simulink model "clustercar8"  (R2016a)
settings: Solver=ode45  StartTime=0.0  StopTime=10.0  MaxStep=0.001  RelTol=1e-3
InitFcn:
  | clc;
  | clear;
  | R = 1/2;
  | L = 1;
  | L1 = [-1 0 1;1 -1 0;0 1 -1];
  | 
  | gammar = 0.75;
  | L1 = [L1,gammar*L1];
  | Vx = [0 0 0]';
  | Vy = [0 0 0];
  | Xend = [3 4 5]';
  | Yend = [3 4 5]';
StopFcn:
  | hold off
  | plot(xx(:,1),xx(:,2),'r',xx(:,3),xx(:,4),'b',xx(:,5),xx(:,6),'g');
  | hold on
  | grid on
  | plot(ss(:,1),ss(:,4),'k--',ss(:,2),ss(:,5),'c--',ss(:,3),ss(:,6),'m--');
libraries: simulink x3
settings Model: Creator=Administrator  LastModifiedBy=Administrator

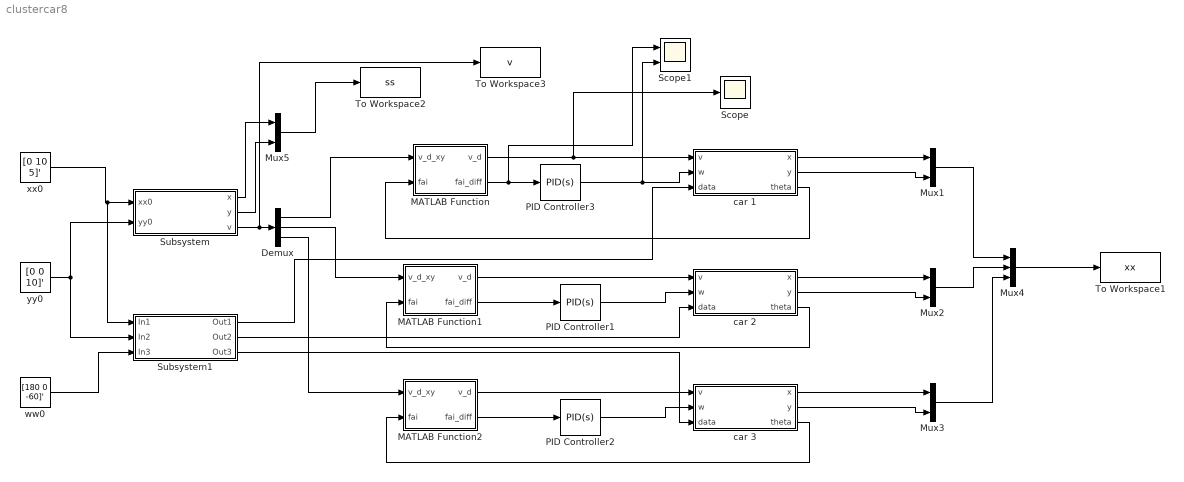
== system clustercar8 ==
  Demux : Demux  Outputs=3
  MATLAB Function : MATLAB Function  TreatAsAtomicUnit=on
  MATLAB Function1 : MATLAB Function  TreatAsAtomicUnit=on
  MATLAB Function2 : MATLAB Function  TreatAsAtomicUnit=on
  Mux{1..3,5} (4 alike) : Mux  Inputs=2
  Mux4 : Mux  Inputs=3
  PID Controller1 : simulink/Continuous/PID Controller  Controller=PID  TimeDomain=Continuous-time  SampleTime=-1  IntegratorMethod=Forward Euler  FilterMethod=Forward Euler  Form=Parallel  UseFilter=on  ControllerParametersSource=internal  P=100  I=10  D=0.01  N=100  InitialConditionSource=internal  InitialConditionForIntegrator=0  InitialConditionForFilter=0  ExternalReset=none  LimitOutput=off  UpperSaturationLimit=inf  LowerSaturationLimit=-inf  LinearizeAsGain=on  AntiWindupMode=none  Kb=1  TrackingMode=off  Kt=1  PParamMin=[]  PParamMax=[]  IParamMin=[]  IParamMax=[]  DParamMin=[]  DParamMax=[]  NParamMin=[]  NParamMax=[]  KbParamMin=[]  KbParamMax=[]  KtParamMin=[]  KtParamMax=[]  POutMin=[]  POutMax=[]  IOutMin=[]  IOutMax=[]  DOutMin=[]  DOutMax=[]  NOutMin=[]  NOutMax=[]  KbOutMin=[]  KbOutMax=[]  KtOutMin=[]  KtOutMax=[]  IntegratorOutMin=[]  IntegratorOutMax=[]  FilterOutMin=[]  FilterOutMax=[]  SumOutMin=[]  SumOutMax=[]  SumI1OutMin=[]  SumI1OutMax=[]  SumI2OutMin=[]  SumI2OutMax=[]  SumI3OutMin=[]  SumI3OutMax=[]  SumDOutMin=[]  SumDOutMax=[]  SaturationOutMin=[]  SaturationOutMax=[]  IntegratorContinuousStateAttributes=''  IntegratorStateMustResolveToSignalObject=off  IntegratorRTWStateStorageClass=Auto  FilterContinuousStateAttributes=''  FilterStateMustResolveToSignalObject=off  FilterRTWStateStorageClass=Auto  DifferentiatorICPrevScaledInput=0  DifferentiatorOutMin=[]  DifferentiatorOutMax=[]
  PID Controller2 : simulink/Continuous/PID Controller  Controller=PID  TimeDomain=Continuous-time  SampleTime=-1  IntegratorMethod=Forward Euler  FilterMethod=Forward Euler  Form=Parallel  UseFilter=on  ControllerParametersSource=internal  P=500  I=10  D=0.01  N=100  InitialConditionSource=internal  InitialConditionForIntegrator=0  InitialConditionForFilter=0  ExternalReset=none  LimitOutput=off  UpperSaturationLimit=inf  LowerSaturationLimit=-inf  LinearizeAsGain=on  AntiWindupMode=none  Kb=1  TrackingMode=off  Kt=1  PParamMin=[]  PParamMax=[]  IParamMin=[]  IParamMax=[]  DParamMin=[]  DParamMax=[]  NParamMin=[]  NParamMax=[]  KbParamMin=[]  KbParamMax=[]  KtParamMin=[]  KtParamMax=[]  POutMin=[]  POutMax=[]  IOutMin=[]  IOutMax=[]  DOutMin=[]  DOutMax=[]  NOutMin=[]  NOutMax=[]  KbOutMin=[]  KbOutMax=[]  KtOutMin=[]  KtOutMax=[]  IntegratorOutMin=[]  IntegratorOutMax=[]  FilterOutMin=[]  FilterOutMax=[]  SumOutMin=[]  SumOutMax=[]  SumI1OutMin=[]  SumI1OutMax=[]  SumI2OutMin=[]  SumI2OutMax=[]  SumI3OutMin=[]  SumI3OutMax=[]  SumDOutMin=[]  SumDOutMax=[]  SaturationOutMin=[]  SaturationOutMax=[]  IntegratorContinuousStateAttributes=''  IntegratorStateMustResolveToSignalObject=off  IntegratorRTWStateStorageClass=Auto  FilterContinuousStateAttributes=''  FilterStateMustResolveToSignalObject=off  FilterRTWStateStorageClass=Auto  DifferentiatorICPrevScaledInput=0  DifferentiatorOutMin=[]  DifferentiatorOutMax=[]
  PID Controller3 : simulink/Continuous/PID Controller  Controller=PID  TimeDomain=Continuous-time  SampleTime=-1  IntegratorMethod=Forward Euler  FilterMethod=Forward Euler  Form=Parallel  UseFilter=on  ControllerParametersSource=internal  P=100  I=10  D=0.01  N=100  InitialConditionSource=internal  InitialConditionForIntegrator=0  InitialConditionForFilter=0  ExternalReset=none  LimitOutput=off  UpperSaturationLimit=inf  LowerSaturationLimit=-inf  LinearizeAsGain=on  AntiWindupMode=none  Kb=1  TrackingMode=off  Kt=1  PParamMin=[]  PParamMax=[]  IParamMin=[]  IParamMax=[]  DParamMin=[]  DParamMax=[]  NParamMin=[]  NParamMax=[]  KbParamMin=[]  KbParamMax=[]  KtParamMin=[]  KtParamMax=[]  POutMin=[]  POutMax=[]  IOutMin=[]  IOutMax=[]  DOutMin=[]  DOutMax=[]  NOutMin=[]  NOutMax=[]  KbOutMin=[]  KbOutMax=[]  KtOutMin=[]  KtOutMax=[]  IntegratorOutMin=[]  IntegratorOutMax=[]  FilterOutMin=[]  FilterOutMax=[]  SumOutMin=[]  SumOutMax=[]  SumI1OutMin=[]  SumI1OutMax=[]  SumI2OutMin=[]  SumI2OutMax=[]  SumI3OutMin=[]  SumI3OutMax=[]  SumDOutMin=[]  SumDOutMax=[]  SaturationOutMin=[]  SaturationOutMax=[]  IntegratorContinuousStateAttributes=''  IntegratorStateMustResolveToSignalObject=off  IntegratorRTWStateStorageClass=Auto  FilterContinuousStateAttributes=''  FilterStateMustResolveToSignalObject=off  FilterRTWStateStorageClass=Auto  DifferentiatorICPrevScaledInput=0  DifferentiatorOutMin=[]  DifferentiatorOutMax=[]
  Scope : Scope
  Scope1 : Scope  NumInputPorts=2
  Subsystem : Subsystem
  Subsystem1 : Subsystem
  To Workspace1 : ToWorkspace  VariableName=xx  SampleTime=-1
  To Workspace2 : ToWorkspace  VariableName=ss  SampleTime=-1
  To Workspace3 : ToWorkspace  VariableName=v  SampleTime=-1
  car 1 : Subsystem
  car 2 : Subsystem
  car 3 : Subsystem
  ww0 : Constant  Value=[180 0 -60]'
  xx0 : Constant  Value=[0 10 5]'
  yy0 : Constant  Value=[0 0 10]'
  wires:
  car 1/1(x) -> Mux1/1
  car 1/2(y) -> Mux1/2
  xx0/1 -> Subsystem1/1(In1), Subsystem/1(xx0)
  yy0/1 -> Subsystem/2(yy0), Subsystem1/2(In2)
  PID Controller1/1 -> car 2/2(w)
  MATLAB Function1/2(fai_diff) -> PID Controller1/1
  MATLAB Function1/1(v_d) -> car 2/1(v)
  PID Controller2/1 -> car 3/2(w)
  MATLAB Function2/2(fai_diff) -> PID Controller2/1
  MATLAB Function2/1(v_d) -> car 3/1(v)
  Subsystem/3(v) -> To Workspace3/1, Demux/1
  Demux/1 -> MATLAB Function/1(v_d_xy)
  Demux/2 -> MATLAB Function1/1(v_d_xy)
  Demux/3 -> MATLAB Function2/1(v_d_xy)
  car 2/1(x) -> Mux2/1
  car 2/2(y) -> Mux2/2
  car 3/1(x) -> Mux3/1
  car 3/2(y) -> Mux3/2
  car 1/3(theta) -> MATLAB Function/2(fai)
  car 2/3(theta) -> MATLAB Function1/2(fai)
  car 3/3(theta) -> MATLAB Function2/2(fai)
  Mux1/1 -> Mux4/1
  Mux2/1 -> Mux4/2
  Mux3/1 -> Mux4/3
  Mux4/1 -> To Workspace1/1
  Subsystem1/1(Out1) -> car 1/3(data)
  Subsystem1/2(Out2) -> car 2/3(data)
  Subsystem1/3(Out3) -> car 3/3(data)
  Mux5/1 -> To Workspace2/1
  Subsystem/1(x) -> Mux5/1
  Subsystem/2(y) -> Mux5/2
  MATLAB Function/1(v_d) -> car 1/1(v), Scope/1
  PID Controller3/1 -> Scope1/2, car 1/2(w)
  ww0/1 -> Subsystem1/3(In3)
  MATLAB Function/2(fai_diff) -> Scope1/1, PID Controller3/1

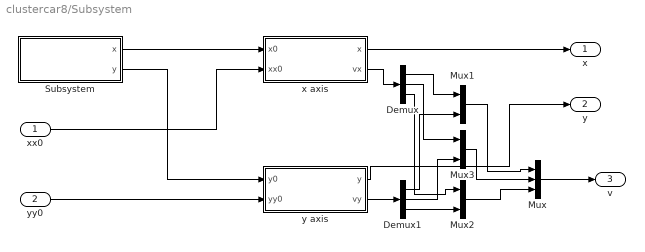
== system clustercar8/Subsystem ==
  xx0 : Inport
  yy0 : Inport  Port=2
  Demux : Demux  Outputs=3
  Demux1 : Demux  Outputs=3
  Mux : Mux  Inputs=3
  Mux1 : Mux  Inputs=2
  Mux2 : Mux  Inputs=2
  Mux3 : Mux  Inputs=2
  Subsystem : Subsystem
  x axis : Subsystem
  y axis : Subsystem
  x : Outport
  y : Outport  Port=2
  v : Outport  Port=3
  wires:
  Subsystem/1(x) -> x axis/1(x0)
  x axis/1(x) -> x/1
  y axis/1(y) -> y/1
  Subsystem/2(y) -> y axis/1(y0)
  Mux/1 -> v/1
  xx0/1 -> x axis/2(xx0)
  yy0/1 -> y axis/2(yy0)
  x axis/2(vx) -> Demux/1
  Demux/1 -> Mux1/1
  Demux/2 -> Mux3/1
  Demux/3 -> Mux2/1
  Demux1/1 -> Mux1/2
  Demux1/2 -> Mux3/2
  Demux1/3 -> Mux2/2
  y axis/2(vy) -> Demux1/1
  Mux1/1 -> Mux/1
  Mux3/1 -> Mux/2
  Mux2/1 -> Mux/3

== system clustercar8/Subsystem1 ==
  In1 : Inport
  In2 : Inport  Port=2
  In3 : Inport  Port=3
  Demux : Demux  Outputs=3
  Demux1 : Demux  Outputs=3
  Demux2 : Demux  Outputs=3
  Gain : Gain  Gain=pi/180
  Mux : Mux  Inputs=3
  Mux1 : Mux  Inputs=3
  Mux2 : Mux  Inputs=3
  Out1 : Outport
  Out2 : Outport  Port=2
  Out3 : Outport  Port=3
  wires:
  In2/1 -> Demux1/1
  In1/1 -> Demux/1
  Demux/1 -> Mux/1
  Demux/2 -> Mux1/1
  Demux/3 -> Mux2/1
  Demux1/1 -> Mux/2
  Demux1/2 -> Mux1/2
  Demux1/3 -> Mux2/2
  Mux/1 -> Out1/1
  Mux1/1 -> Out2/1
  Mux2/1 -> Out3/1
  In3/1 -> Gain/1
  Demux2/1 -> Mux/3
  Demux2/2 -> Mux1/3
  Demux2/3 -> Mux2/3
  Gain/1 -> Demux2/1

== system clustercar8/car 1 ==
  v : Inport
  w : Inport  Port=2
  data : Inport  Port=3
  Subsystem1 : Subsystem
  Subsystem2 : Subsystem
  x : Outport
  y : Outport  Port=2
  theta : Outport  Port=3
  wires:
  Subsystem1/1(vr) -> Subsystem2/1("vr ")
  Subsystem1/2(vl) -> Subsystem2/2("vl ")
  w/1 -> Subsystem1/2(w)
  v/1 -> Subsystem1/1(v)
  data/1 -> Subsystem2/3(data)
  Subsystem2/1(x) -> x/1
  Subsystem2/2(y) -> y/1
  Subsystem2/3(theta) -> theta/1

== system clustercar8/car 2 ==
  v : Inport
  w : Inport  Port=2
  data : Inport  Port=3
  Subsystem1 : Subsystem
  Subsystem2 : Subsystem
  x : Outport
  y : Outport  Port=2
  theta : Outport  Port=3
  wires:
  Subsystem1/1(vr) -> Subsystem2/1("vr ")
  Subsystem1/2(vl) -> Subsystem2/2("vl ")
  w/1 -> Subsystem1/2(w)
  v/1 -> Subsystem1/1(v)
  data/1 -> Subsystem2/3(data)
  Subsystem2/1(x) -> x/1
  Subsystem2/2(y) -> y/1
  Subsystem2/3(theta) -> theta/1

== system clustercar8/car 3 ==
  v : Inport
  w : Inport  Port=2
  data : Inport  Port=3
  Subsystem1 : Subsystem
  Subsystem2 : Subsystem
  x : Outport
  y : Outport  Port=2
  theta : Outport  Port=3
  wires:
  Subsystem1/1(vr) -> Subsystem2/1("vr ")
  Subsystem1/2(vl) -> Subsystem2/2("vl ")
  w/1 -> Subsystem1/2(w)
  v/1 -> Subsystem1/1(v)
  data/1 -> Subsystem2/3(data)
  Subsystem2/1(x) -> x/1
  Subsystem2/2(y) -> y/1
  Subsystem2/3(theta) -> theta/1

== system clustercar8/Subsystem/Subsystem ==
  三角形path : Subsystem
  圆 : Subsystem
  日地月 : Subsystem
  点 : Subsystem
  x : Outport
  y : Outport  Port=2
  wires:
  日地月/1(x) -> x/1
  日地月/2(y) -> y/1

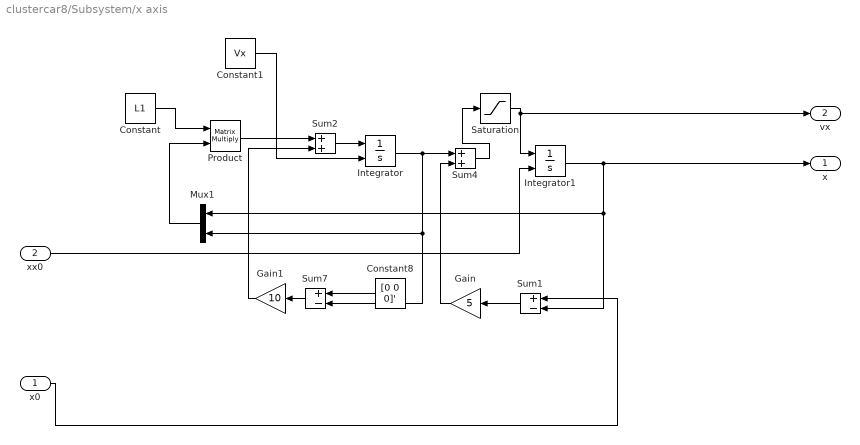
== system clustercar8/Subsystem/x axis ==
  x0 : Inport
  xx0 : Inport  Port=2
  Constant : Constant  Value=L1  VectorParams1D=off
  Constant1 : Constant  Value=Vx
  Constant8 : Constant  Value=[0 0 0]'
  Gain : Gain  Gain=5
  Gain1 : Gain  Gain=10
  Integrator : Integrator  InitialConditionSource=external
  Integrator1 : Integrator  InitialConditionSource=external
  Mux1 : Mux  Inputs=2
  Product : Product  Multiplication=Matrix(*)
  Saturation : Saturate  UpperLimit=5  LowerLimit=-5
  Sum1 : Sum  Inputs=+-
  Sum2 : Sum
  Sum4 : Sum
  Sum7 : Sum  Inputs=+-
  x : Outport
  vx : Outport  Port=2
  wires:
  Constant/1 -> Product/1
  Constant1/1 -> Integrator/2
  xx0/1 -> Integrator1/2
  Mux1/1 -> Product/2
  Product/1 -> Sum2/1
  Sum2/1 -> Integrator/1
  Integrator/1 -> Sum4/1, Sum7/2, Mux1/2
  Constant8/1 -> Sum7/1
  Sum7/1 -> Gain1/1
  Gain1/1 -> Sum2/2
  x0/1 -> Sum1/1
  Integrator1/1 -> x/1, Sum1/2, Mux1/1
  Sum1/1 -> Gain/1
  Gain/1 -> Sum4/2
  Sum4/1 -> Saturation/1
  Saturation/1 -> Integrator1/1, vx/1

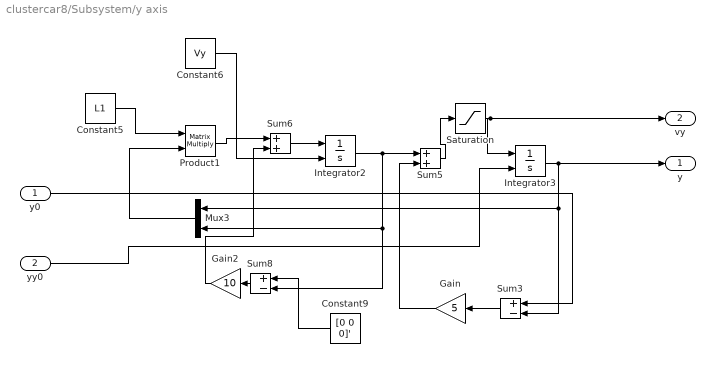
== system clustercar8/Subsystem/y axis ==
  y0 : Inport
  yy0 : Inport  Port=2
  Constant5 : Constant  Value=L1  VectorParams1D=off
  Constant6 : Constant  Value=Vy
  Constant9 : Constant  Value=[0 0 0]'
  Gain : Gain  Gain=5
  Gain2 : Gain  Gain=10
  Integrator2 : Integrator  InitialConditionSource=external
  Integrator3 : Integrator  InitialConditionSource=external
  Mux3 : Mux  Inputs=2
  Product1 : Product  Multiplication=Matrix(*)
  Saturation : Saturate  UpperLimit=5  LowerLimit=-5
  Sum3 : Sum  Inputs=+-
  Sum5 : Sum
  Sum6 : Sum
  Sum8 : Sum  Inputs=+-
  y : Outport
  vy : Outport  Port=2
  wires:
  Constant5/1 -> Product1/1
  Constant6/1 -> Integrator2/2
  yy0/1 -> Integrator3/2
  Integrator3/1 -> y/1, Sum3/2, Mux3/1
  Mux3/1 -> Product1/2
  Product1/1 -> Sum6/1
  Sum6/1 -> Integrator2/1
  Integrator2/1 -> Sum8/2, Mux3/2, Sum5/1
  Constant9/1 -> Sum8/1
  Sum8/1 -> Gain2/1
  Sum3/1 -> Gain/1
  Gain/1 -> Sum5/2
  Gain2/1 -> Sum6/2
  y0/1 -> Sum3/1
  Saturation/1 -> Integrator3/1, vy/1
  Sum5/1 -> Saturation/1

== system clustercar8/car 1/Subsystem1 ==
  v : Inport
  w : Inport  Port=2
  Demux : Demux  Outputs=2
  Matrix Multiply : Product  Multiplication=Matrix(*)
  Mux : Mux  Inputs=2
  R + L : Constant  Value=[1/R,L/(2*R);1/R,-L/(2*R)]
  vr : Outport
  vl : Outport  Port=2
  wires:
  v/1 -> Mux/1
  w/1 -> Mux/2
  Mux/1 -> Matrix Multiply/2
  Matrix Multiply/1 -> Demux/1
  Demux/1 -> vr/1
  Demux/2 -> vl/1
  R + L/1 -> Matrix Multiply/1

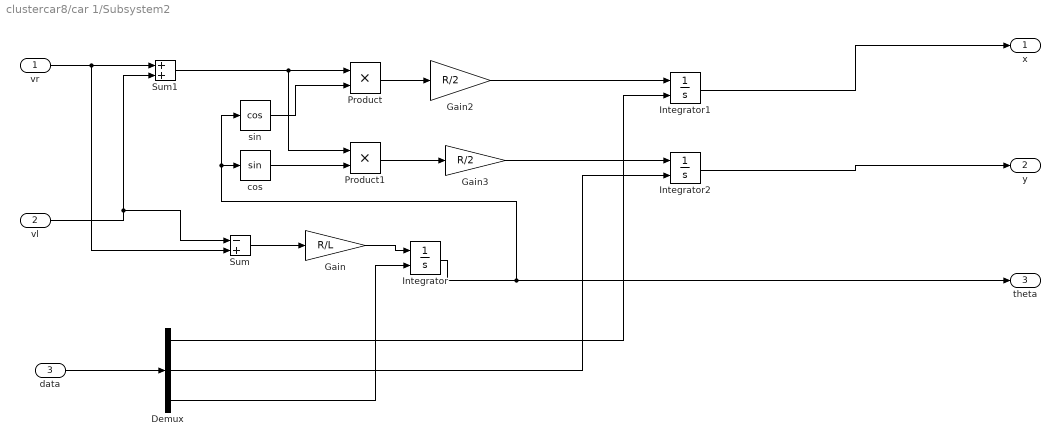
== system clustercar8/car 1/Subsystem2 ==
  "vr " : Inport
  "vl " : Inport  Port=2
  data : Inport  Port=3
  Demux : Demux  Outputs=3
  Gain : Gain  Gain=R/L
  Gain2 : Gain  Gain=R/2
  Gain3 : Gain  Gain=R/2
  Integrator : Integrator  InitialConditionSource=external
  Integrator1 : Integrator  InitialConditionSource=external
  Integrator2 : Integrator  InitialConditionSource=external
  Product : Product
  Product1 : Product
  Sum : Sum  Inputs=-+
  Sum1 : Sum
  cos : Trigonometry
  sin : Trigonometry  Operator=cos
  x : Outport
  y : Outport  Port=2
  theta : Outport  Port=3
  wires:
  "vl "/1 -> Sum1/2, Sum/1
  "vr "/1 -> Sum/2, Sum1/1
  Sum/1 -> Gain/1
  Gain/1 -> Integrator/1
  Integrator/1 -> theta/1, sin/1, cos/1
  Sum1/1 -> Product1/1, Product/1
  sin/1 -> Product/2
  cos/1 -> Product1/2
  Product/1 -> Gain2/1
  Product1/1 -> Gain3/1
  Gain2/1 -> Integrator1/1
  Gain3/1 -> Integrator2/1
  Integrator1/1 -> x/1
  Integrator2/1 -> y/1
  data/1 -> Demux/1
  Demux/1 -> Integrator1/2
  Demux/2 -> Integrator2/2
  Demux/3 -> Integrator/2

== system clustercar8/car 2/Subsystem1 ==
  v : Inport
  w : Inport  Port=2
  Demux : Demux  Outputs=2
  Matrix Multiply : Product  Multiplication=Matrix(*)
  Mux : Mux  Inputs=2
  R + L : Constant  Value=[1/R,L/(2*R);1/R,-L/(2*R)]
  vr : Outport
  vl : Outport  Port=2
  wires:
  v/1 -> Mux/1
  w/1 -> Mux/2
  Mux/1 -> Matrix Multiply/2
  Matrix Multiply/1 -> Demux/1
  Demux/1 -> vr/1
  Demux/2 -> vl/1
  R + L/1 -> Matrix Multiply/1

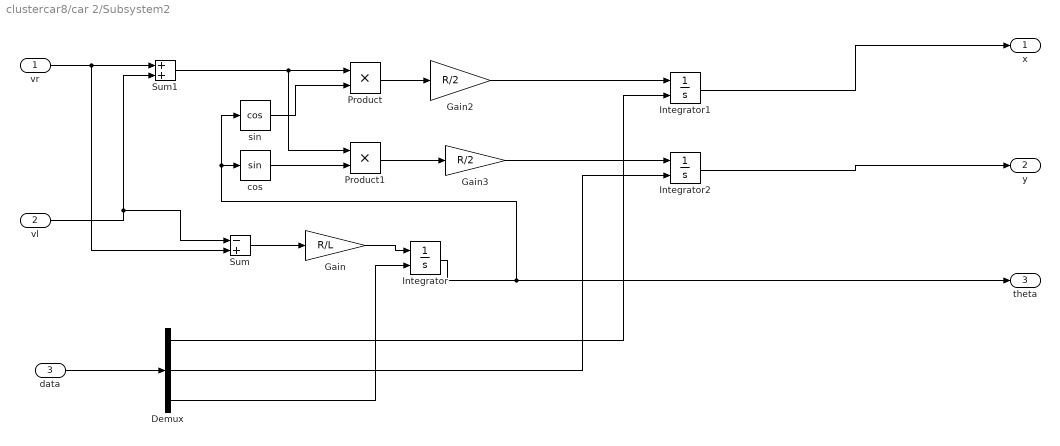
== system clustercar8/car 2/Subsystem2 ==
  "vr " : Inport
  "vl " : Inport  Port=2
  data : Inport  Port=3
  Demux : Demux  Outputs=3
  Gain : Gain  Gain=R/L
  Gain2 : Gain  Gain=R/2
  Gain3 : Gain  Gain=R/2
  Integrator : Integrator  InitialConditionSource=external
  Integrator1 : Integrator  InitialConditionSource=external
  Integrator2 : Integrator  InitialConditionSource=external
  Product : Product
  Product1 : Product
  Sum : Sum  Inputs=-+
  Sum1 : Sum
  cos : Trigonometry
  sin : Trigonometry  Operator=cos
  x : Outport
  y : Outport  Port=2
  theta : Outport  Port=3
  wires:
  "vl "/1 -> Sum1/2, Sum/1
  "vr "/1 -> Sum/2, Sum1/1
  Sum/1 -> Gain/1
  Gain/1 -> Integrator/1
  Integrator/1 -> theta/1, sin/1, cos/1
  Sum1/1 -> Product1/1, Product/1
  sin/1 -> Product/2
  cos/1 -> Product1/2
  Product/1 -> Gain2/1
  Product1/1 -> Gain3/1
  Gain2/1 -> Integrator1/1
  Gain3/1 -> Integrator2/1
  Integrator1/1 -> x/1
  Integrator2/1 -> y/1
  data/1 -> Demux/1
  Demux/1 -> Integrator1/2
  Demux/2 -> Integrator2/2
  Demux/3 -> Integrator/2

== system clustercar8/car 3/Subsystem1 ==
  v : Inport
  w : Inport  Port=2
  Demux : Demux  Outputs=2
  Matrix Multiply : Product  Multiplication=Matrix(*)
  Mux : Mux  Inputs=2
  R + L : Constant  Value=[1/R,L/(2*R);1/R,-L/(2*R)]
  vr : Outport
  vl : Outport  Port=2
  wires:
  v/1 -> Mux/1
  w/1 -> Mux/2
  Mux/1 -> Matrix Multiply/2
  Matrix Multiply/1 -> Demux/1
  Demux/1 -> vr/1
  Demux/2 -> vl/1
  R + L/1 -> Matrix Multiply/1

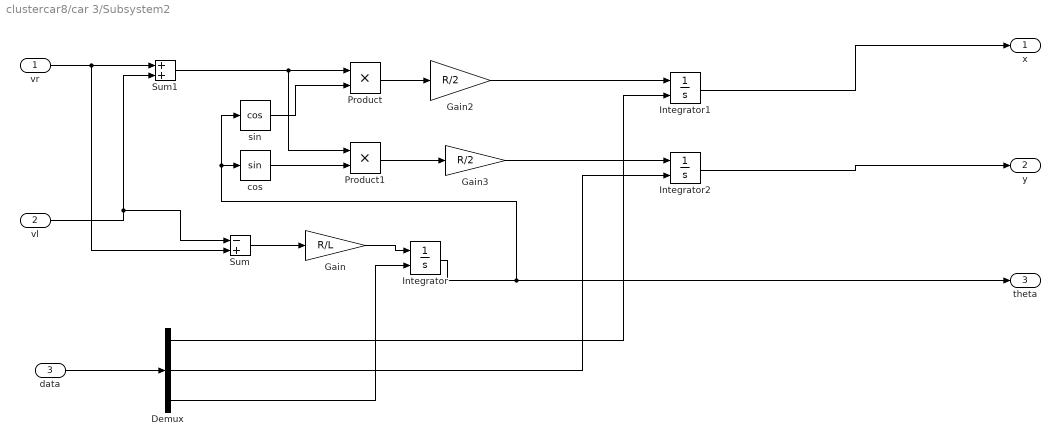
== system clustercar8/car 3/Subsystem2 ==
  "vr " : Inport
  "vl " : Inport  Port=2
  data : Inport  Port=3
  Demux : Demux  Outputs=3
  Gain : Gain  Gain=R/L
  Gain2 : Gain  Gain=R/2
  Gain3 : Gain  Gain=R/2
  Integrator : Integrator  InitialConditionSource=external
  Integrator1 : Integrator  InitialConditionSource=external
  Integrator2 : Integrator  InitialConditionSource=external
  Product : Product
  Product1 : Product
  Sum : Sum  Inputs=-+
  Sum1 : Sum
  cos : Trigonometry
  sin : Trigonometry  Operator=cos
  x : Outport
  y : Outport  Port=2
  theta : Outport  Port=3
  wires:
  "vl "/1 -> Sum1/2, Sum/1
  "vr "/1 -> Sum/2, Sum1/1
  Sum/1 -> Gain/1
  Gain/1 -> Integrator/1
  Integrator/1 -> theta/1, sin/1, cos/1
  Sum1/1 -> Product1/1, Product/1
  sin/1 -> Product/2
  cos/1 -> Product1/2
  Product/1 -> Gain2/1
  Product1/1 -> Gain3/1
  Gain2/1 -> Integrator1/1
  Gain3/1 -> Integrator2/1
  Integrator1/1 -> x/1
  Integrator2/1 -> y/1
  data/1 -> Demux/1
  Demux/1 -> Integrator1/2
  Demux/2 -> Integrator2/2
  Demux/3 -> Integrator/2

== system clustercar8/Subsystem/Subsystem/三角形path ==
  Mux1 : Mux  Inputs=3
  Mux7 : Mux  Inputs=3
  Subsystem1 : Subsystem
  Subsystem3 : Subsystem
  Subsystem5 : Subsystem
  v : DiscretePulseGenerator  PulseType=Time based  Amplitude=5  PulseWidth=50
  v1 : DiscretePulseGenerator  PulseType=Time based  Amplitude=5  PulseWidth=50
  v2 : DiscretePulseGenerator  PulseType=Time based  Amplitude=5  PulseWidth=50
  w : DiscretePulseGenerator  PulseType=Time based  Amplitude=2*pi/3  PulseWidth=50  PhaseDelay=1
  w1 : DiscretePulseGenerator  PulseType=Time based  Amplitude=2*pi/3  PulseWidth=50  PhaseDelay=1
  w2 : DiscretePulseGenerator  PulseType=Time based  Amplitude=2*pi/3  PulseWidth=50  PhaseDelay=1
  x : Outport
  y : Outport  Port=2
  wires:
  Subsystem1/1(x) -> Mux7/1
  v/1 -> Subsystem1/1(v)
  w/1 -> Subsystem1/2(w)
  v1/1 -> Subsystem3/1(v)
  w1/1 -> Subsystem3/2(w)
  v2/1 -> Subsystem5/1(v)
  w2/1 -> Subsystem5/2(w)
  Subsystem3/1(x) -> Mux7/2
  Subsystem5/1(x) -> Mux7/3
  Subsystem1/2(y) -> Mux1/1
  Subsystem3/2(y) -> Mux1/2
  Subsystem5/2(y) -> Mux1/3
  Mux7/1 -> x/1
  Mux1/1 -> y/1

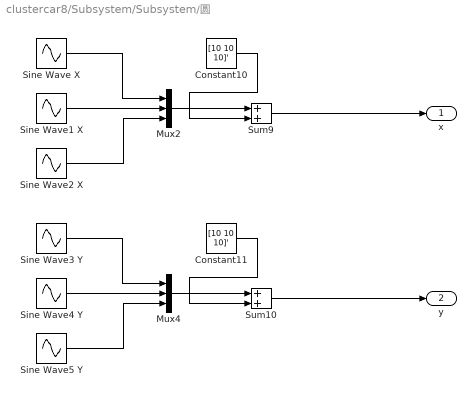
== system clustercar8/Subsystem/Subsystem/圆 ==
  Constant10 : Constant  Value=[10 10 10]'
  Constant11 : Constant  Value=[10 10 10]'
  Mux2 : Mux  Inputs=3
  Mux4 : Mux  Inputs=3
  Sine Wave X : Sin  Amplitude=2  SampleTime=0
  Sine Wave1 X : Sin  Amplitude=2  Phase=120*pi/180  SampleTime=0
  Sine Wave2 X : Sin  Amplitude=2  Phase=240*pi/180  SampleTime=0
  Sine Wave3 Y : Sin  Amplitude=2  Phase=90*pi/180  SampleTime=0
  Sine Wave4 Y : Sin  Amplitude=2  Phase=210*pi/180  SampleTime=0
  Sine Wave5 Y : Sin  Amplitude=2  Phase=330*pi/180  SampleTime=0
  Sum10 : Sum
  Sum9 : Sum
  x : Outport
  y : Outport  Port=2
  wires:
  Sine Wave X/1 -> Mux2/1
  Sine Wave1 X/1 -> Mux2/2
  Sine Wave2 X/1 -> Mux2/3
  Mux2/1 -> Sum9/1
  Constant10/1 -> Sum9/2
  Sine Wave3 Y/1 -> Mux4/1
  Sine Wave4 Y/1 -> Mux4/2
  Sine Wave5 Y/1 -> Mux4/3
  Mux4/1 -> Sum10/1
  Constant11/1 -> Sum10/2
  Sum10/1 -> y/1
  Sum9/1 -> x/1

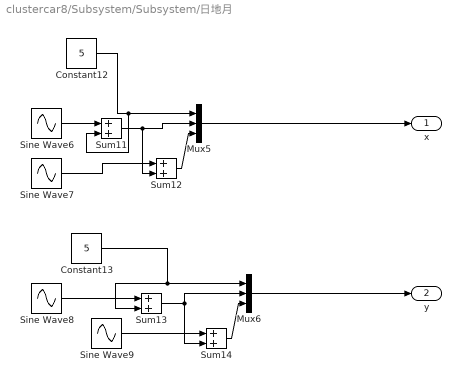
== system clustercar8/Subsystem/Subsystem/日地月 ==
  Constant12 : Constant  Value=5
  Constant13 : Constant  Value=5
  Mux5 : Mux  Inputs=3
  Mux6 : Mux  Inputs=3
  Sine Wave6 : Sin  Amplitude=2  SampleTime=0
  Sine Wave7 : Sin  Amplitude=0.5  Frequency=20  SampleTime=0
  Sine Wave8 : Sin  Amplitude=2  Phase=90*pi/180  SampleTime=0
  Sine Wave9 : Sin  Amplitude=0.5  Frequency=20  Phase=90*pi/180  SampleTime=0
  Sum{11..14} (4 alike) : Sum
  x : Outport
  y : Outport  Port=2
  wires:
  Constant12/1 -> Mux5/1, Sum11/2
  Sine Wave6/1 -> Sum11/1
  Sine Wave7/1 -> Sum12/1
  Sum12/1 -> Mux5/3
  Sum11/1 -> Sum12/2, Mux5/2
  Constant13/1 -> Mux6/1, Sum13/2
  Sine Wave8/1 -> Sum13/1
  Sum13/1 -> Mux6/2, Sum14/2
  Sine Wave9/1 -> Sum14/1
  Sum14/1 -> Mux6/3
  Mux5/1 -> x/1
  Mux6/1 -> y/1

== system clustercar8/Subsystem/Subsystem/点 ==
  Constant3 : Constant  Value=Xend
  Constant4 : Constant  Value=Yend
  x : Outport
  y : Outport  Port=2
  wires:
  Constant3/1 -> x/1
  Constant4/1 -> y/1

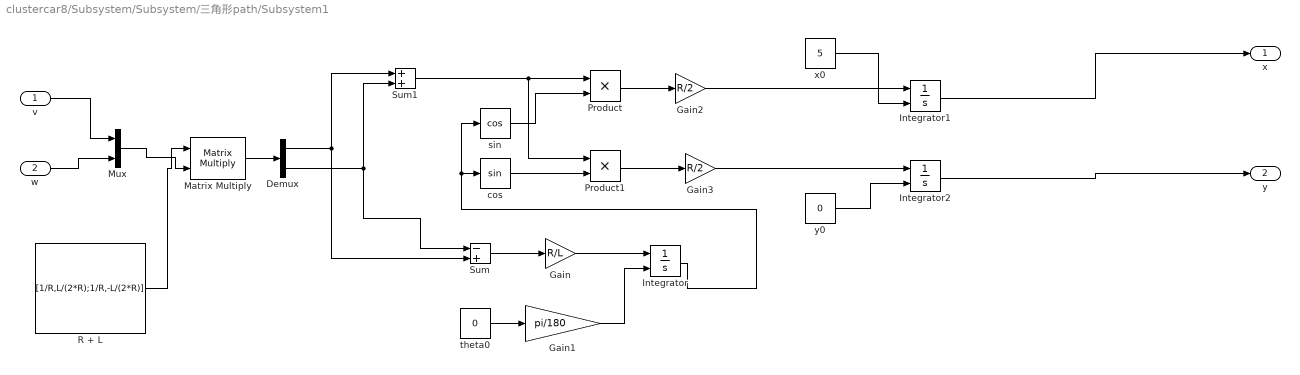
== system clustercar8/Subsystem/Subsystem/三角形path/Subsystem1 ==
  v : Inport
  w : Inport  Port=2
  Demux : Demux  Outputs=2
  Gain : Gain  Gain=R/L
  Gain1 : Gain  Gain=pi/180
  Gain2 : Gain  Gain=R/2
  Gain3 : Gain  Gain=R/2
  Integrator : Integrator  InitialConditionSource=external
  Integrator1 : Integrator  InitialConditionSource=external
  Integrator2 : Integrator  InitialConditionSource=external
  Matrix Multiply : Product  Multiplication=Matrix(*)
  Mux : Mux  Inputs=2
  Product : Product
  Product1 : Product
  R + L : Constant  Value=[1/R,L/(2*R);1/R,-L/(2*R)]
  Sum : Sum  Inputs=-+
  Sum1 : Sum
  cos : Trigonometry
  sin : Trigonometry  Operator=cos
  theta0 : Constant  Value=0
  x0 : Constant  Value=5
  y0 : Constant  Value=0
  x : Outport
  y : Outport  Port=2
  wires:
  Demux/2 -> Sum/1, Sum1/2
  Demux/1 -> Sum1/1, Sum/2
  Sum/1 -> Gain/1
  Gain/1 -> Integrator/1
  Integrator/1 -> sin/1, cos/1
  theta0/1 -> Gain1/1
  Gain1/1 -> Integrator/2
  Sum1/1 -> Product1/1, Product/1
  sin/1 -> Product/2
  cos/1 -> Product1/2
  Product/1 -> Gain2/1
  Product1/1 -> Gain3/1
  Gain2/1 -> Integrator1/1
  Gain3/1 -> Integrator2/1
  y0/1 -> Integrator2/2
  x0/1 -> Integrator1/2
  Integrator1/1 -> x/1
  Integrator2/1 -> y/1
  v/1 -> Mux/1
  w/1 -> Mux/2
  Mux/1 -> Matrix Multiply/2
  Matrix Multiply/1 -> Demux/1
  R + L/1 -> Matrix Multiply/1

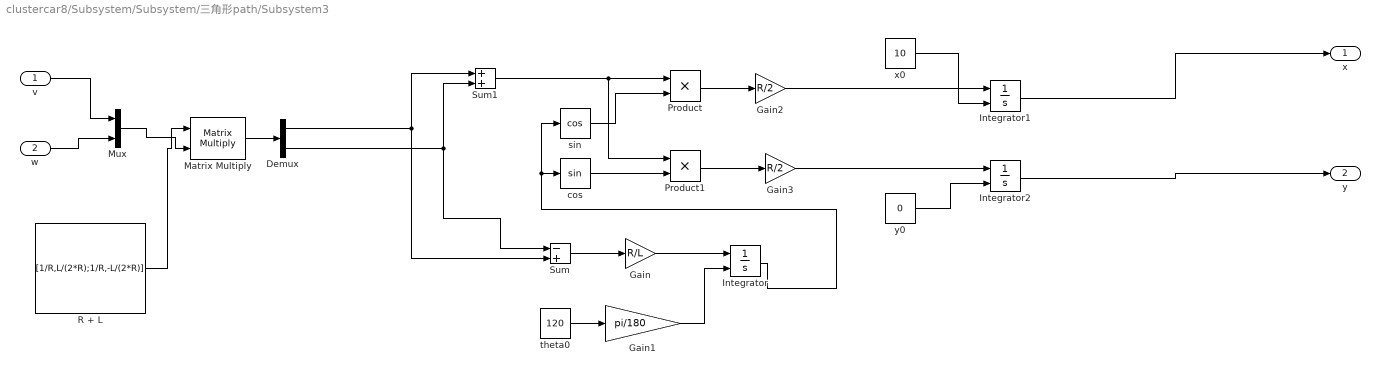
== system clustercar8/Subsystem/Subsystem/三角形path/Subsystem3 ==
  v : Inport
  w : Inport  Port=2
  Demux : Demux  Outputs=2
  Gain : Gain  Gain=R/L
  Gain1 : Gain  Gain=pi/180
  Gain2 : Gain  Gain=R/2
  Gain3 : Gain  Gain=R/2
  Integrator : Integrator  InitialConditionSource=external
  Integrator1 : Integrator  InitialConditionSource=external
  Integrator2 : Integrator  InitialConditionSource=external
  Matrix Multiply : Product  Multiplication=Matrix(*)
  Mux : Mux  Inputs=2
  Product : Product
  Product1 : Product
  R + L : Constant  Value=[1/R,L/(2*R);1/R,-L/(2*R)]
  Sum : Sum  Inputs=-+
  Sum1 : Sum
  cos : Trigonometry
  sin : Trigonometry  Operator=cos
  theta0 : Constant  Value=120
  x0 : Constant  Value=10
  y0 : Constant  Value=0
  x : Outport
  y : Outport  Port=2
  wires:
  Demux/2 -> Sum/1, Sum1/2
  Demux/1 -> Sum1/1, Sum/2
  Sum/1 -> Gain/1
  Gain/1 -> Integrator/1
  Integrator/1 -> sin/1, cos/1
  theta0/1 -> Gain1/1
  Gain1/1 -> Integrator/2
  Sum1/1 -> Product1/1, Product/1
  sin/1 -> Product/2
  cos/1 -> Product1/2
  Product/1 -> Gain2/1
  Product1/1 -> Gain3/1
  Gain2/1 -> Integrator1/1
  Gain3/1 -> Integrator2/1
  y0/1 -> Integrator2/2
  x0/1 -> Integrator1/2
  Integrator1/1 -> x/1
  Integrator2/1 -> y/1
  v/1 -> Mux/1
  w/1 -> Mux/2
  Mux/1 -> Matrix Multiply/2
  Matrix Multiply/1 -> Demux/1
  R + L/1 -> Matrix Multiply/1

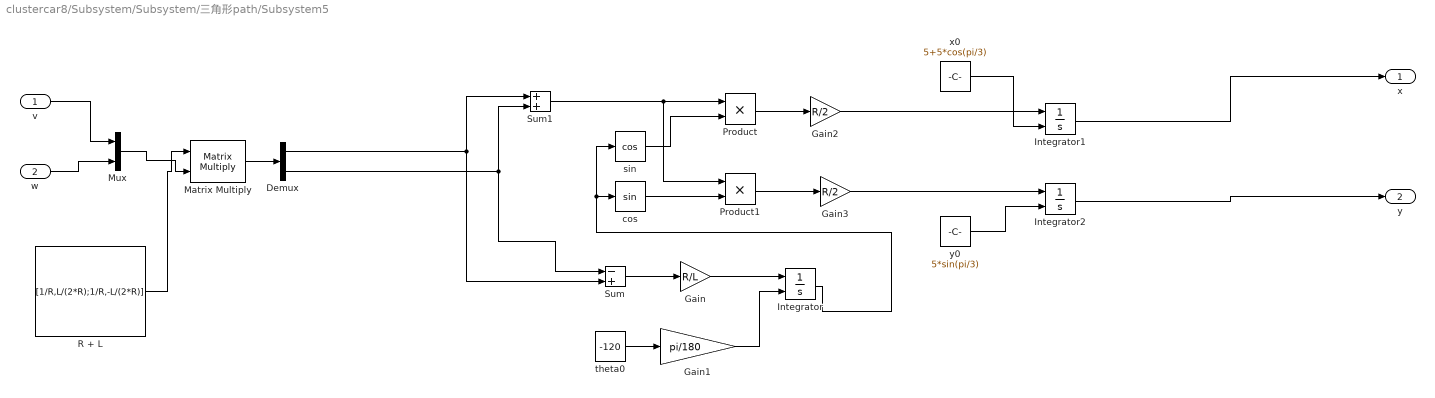
== system clustercar8/Subsystem/Subsystem/三角形path/Subsystem5 ==
  v : Inport
  w : Inport  Port=2
  Demux : Demux  Outputs=2
  Gain : Gain  Gain=R/L
  Gain1 : Gain  Gain=pi/180
  Gain2 : Gain  Gain=R/2
  Gain3 : Gain  Gain=R/2
  Integrator : Integrator  InitialConditionSource=external
  Integrator1 : Integrator  InitialConditionSource=external
  Integrator2 : Integrator  InitialConditionSource=external
  Matrix Multiply : Product  Multiplication=Matrix(*)
  Mux : Mux  Inputs=2
  Product : Product
  Product1 : Product
  R + L : Constant  Value=[1/R,L/(2*R);1/R,-L/(2*R)]
  Sum : Sum  Inputs=-+
  Sum1 : Sum
  cos : Trigonometry
  sin : Trigonometry  Operator=cos
  theta0 : Constant  Value=-120
  x0 : Constant  Value=5+5*cos(pi/3)
  y0 : Constant  Value=5*sin(pi/3)
  x : Outport
  y : Outport  Port=2
  wires:
  Demux/2 -> Sum/1, Sum1/2
  Demux/1 -> Sum1/1, Sum/2
  Sum/1 -> Gain/1
  Gain/1 -> Integrator/1
  Integrator/1 -> sin/1, cos/1
  theta0/1 -> Gain1/1
  Gain1/1 -> Integrator/2
  Sum1/1 -> Product1/1, Product/1
  sin/1 -> Product/2
  cos/1 -> Product1/2
  Product/1 -> Gain2/1
  Product1/1 -> Gain3/1
  Gain2/1 -> Integrator1/1
  Gain3/1 -> Integrator2/1
  y0/1 -> Integrator2/2
  x0/1 -> Integrator1/2
  Integrator1/1 -> x/1
  Integrator2/1 -> y/1
  v/1 -> Mux/1
  w/1 -> Mux/2
  Mux/1 -> Matrix Multiply/2
  Matrix Multiply/1 -> Demux/1
  R + L/1 -> Matrix Multiply/1

== matlab function clustercar8/MATLAB Function1 ==
  data: v_d_xy input; v_d output; fai input; fai_diff output
function [v_d,fai_diff]  = fcn(v_d_xy,fai)
%#codegen

%v_d=[0];
%fai_diff=[0];
v_d =0;
fai_diff=0;
fai_d=0;
v_d = sqrt(v_d_xy(1).^2+ v_d_xy(2).^2);
fai_d = atan2(v_d_xy(2),v_d_xy(1));
fai_diff = fai_d-fai;
if fai_diff>pi
    fai_diff=fai_diff-2*pi*round(fai_diff/(2*pi));
elseif fai_diff(1)<-pi
    fai_diff=fai_diff+2*pi*round(fai_diff/(-2*pi));      
end

end

== matlab function clustercar8/MATLAB Function ==
  data: v_d_xy input; v_d output; fai input; fai_diff output
function [v_d,fai_diff]  = fcn(v_d_xy,fai)
%#codegen

%v_d=[0];
%fai_diff=[0];
v_d =0;
fai_diff=0;
fai_d=0;
v_d = sqrt(v_d_xy(1).^2+ v_d_xy(2).^2);
fai_d = atan2(v_d_xy(2),v_d_xy(1));
fai_diff = fai_d-fai;
if fai_diff>pi
    fai_diff=fai_diff-2*pi*round(fai_diff/(2*pi));
elseif fai_diff(1)<-pi
    fai_diff=fai_diff+2*pi*round(fai_diff/(-2*pi));      
end

end

== matlab function clustercar8/MATLAB Function2 ==
  data: v_d_xy input; v_d output; fai input; fai_diff output
function [v_d,fai_diff]  = fcn(v_d_xy,fai)
%#codegen

%v_d=[0];
%fai_diff=[0];
v_d =0;
fai_diff=0;
fai_d=0;
v_d = sqrt(v_d_xy(1).^2+ v_d_xy(2).^2);
fai_d = atan2(v_d_xy(2),v_d_xy(1));
fai_diff = fai_d-fai;
if fai_diff>pi
    fai_diff=fai_diff-2*pi*round(fai_diff/(2*pi));
elseif fai_diff(1)<-pi
    fai_diff=fai_diff+2*pi*round(fai_diff/(-2*pi));      
end

end
